simulink model "s5_2"  (Simulink 6.6)
settings: Solver=ode45  SolverMode=SingleTasking  StartTime=0.0  StopTime=t_d  FixedStep=Tc  MaxStep=Tc  RelTol=1e-8  AbsTol=1e-8
values from neighbouring files (symbols this model uses):
  C_i = 1    [i5_2.m]
  F_m = 0.01    [i5_2.m]
  G_v = 1    [i5_2.m]
  I_m = 0.0014    [i5_2.m]
  k_t = 0.2    [i5_2.m]
  k_v = 0.2    [i5_2.m]
  L_a = 2e-3    (= 0.002)    [i5_2.m]
  R_a = 0.2    [i5_2.m]
  T_v = 0.1e-3    (= 0.0001)    [i5_2.m]
  Ts = 0.001    [i5_2.m]
settings Model: Creator=luigivillani  LastModifiedBy=luigivillani  ExtModeAutoUpdateStatusClock=off
settings SolverCC: InitialStep=0.1*Tc
settings DataIOCC: LimitDataPoints=off  SaveOutput=off  SaveTime=off
settings OptimizationCC: BlockReduction=off  BooleanDataType=off
settings DebuggingCC: SignalResolutionControl=TryResolveAllWithWarning  SolverPrmCheckMsg=none  MultiTaskDSMMsg=warning  MultiTaskCondExecSysMsg=none  StrictBusMsg=None
settings HardwareCC: TargetUnknown=on
settings RTWCC: IncludeERTFirstTime=on

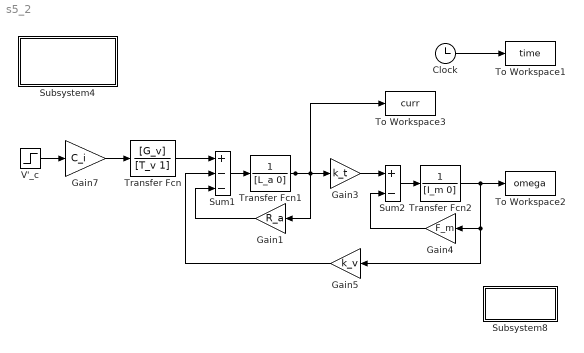
== system s5_2 ==
  Clock : Clock
  Gain1 : Gain  Orientation=left  Gain=R_a  SaturateOnIntegerOverflow=on
      mask Display: disp('R_a')
  Gain3 : Gain  Gain=k_t  SaturateOnIntegerOverflow=on
      mask Display: disp('k_t')
  Gain4 : Gain  Orientation=left  Gain=F_m  SaturateOnIntegerOverflow=on
      mask Display: disp('F_m')
  Gain5 : Gain  Orientation=left  Gain=k_v  SaturateOnIntegerOverflow=on
      mask Display: disp('k_v')
  Gain7 : Gain  Gain=C_i  SaturateOnIntegerOverflow=on
      mask Display: disp('C_i')
  Subsystem4 : Subsystem
      settings: OpenFcn=clear all;i5_2;
      mask Display: disp('variables\ninitialization')
  Subsystem8 : Subsystem  Orientation=left
      settings: OpenFcn=p5_2;
      mask Display: disp('plot')
  Sum1 : Sum  Inputs=+--  SaturateOnIntegerOverflow=on  InputSameDT=on
  Sum2 : Sum  Inputs=+-  SaturateOnIntegerOverflow=on  InputSameDT=on
  To Workspace1 : ToWorkspace  VariableName=time  SampleTime=Ts  SaveFormat=Array
      settings: MaxDataPoints=5001
  To Workspace2 : ToWorkspace  VariableName=omega  SampleTime=Ts  SaveFormat=Array
      settings: MaxDataPoints=5001
  To Workspace3 : ToWorkspace  VariableName=curr  SampleTime=Ts  SaveFormat=Array
      settings: MaxDataPoints=5001
  Transfer Fcn : TransferFcn  Numerator=[G_v]  Denominator=[T_v 1]
  Transfer Fcn1 : TransferFcn  Denominator=[L_a 0]
  Transfer Fcn2 : TransferFcn  Denominator=[I_m 0]
  V'_c : Step  Time=0.0001  SampleTime=0
  wires:
  Gain7/1 -> Transfer Fcn/1
  Transfer Fcn/1 -> Sum1/1
  Sum1/1 -> Transfer Fcn1/1
  Gain3/1 -> Sum2/1
  Sum2/1 -> Transfer Fcn2/1
  Gain4/1 -> Sum2/2
  Transfer Fcn1/1 -> Gain3/1, Gain1/1, To Workspace3/1
  Gain1/1 -> Sum1/3
  Gain5/1 -> Sum1/2
  Clock/1 -> To Workspace1/1
  V'_c/1 -> Gain7/1
  Transfer Fcn2/1 -> To Workspace2/1, Gain4/1, Gain5/1

== system s5_2/Subsystem4 ==
  note: start

== system s5_2/Subsystem8 ==
  note: start
